simulink model "takeoff_sim"  (R2021b)
settings: Solver=VariableStepAuto  StartTime=0.0  StopTime=5  RelTol=1e-3
values from neighbouring files (symbols this model uses):
  A_cxsec = .0166*1.524 + .014    (= 0.0392984)    [Takeoff_Analysis.m]
  C_do = .03    (= 0.03)    [Takeoff_Analysis.m]
  C_L = 1.4    [Takeoff_Analysis.m]
  g = 9.8    [Takeoff_Analysis.m]
  m = 6.35    [Takeoff_Analysis.m]
  mu = 0.015    [Takeoff_Analysis.m]
  rho = 1.225    [Takeoff_Analysis.m]
  S_cref = 0.46    [Takeoff_Analysis.m]
  S_tref = 0.6    [Takeoff_Analysis.m]
settings Model: Creator=medium boss  LastModifiedBy=medium boss

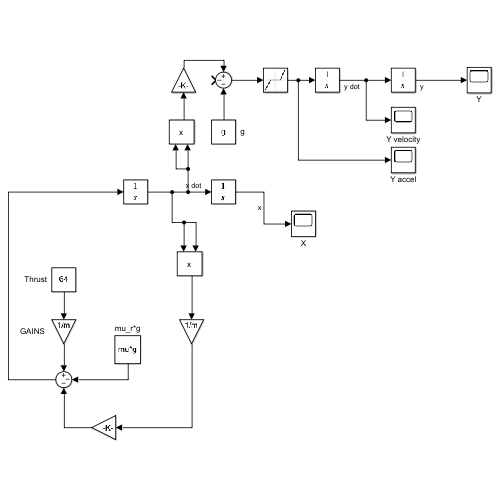
[thumbnail: Simulink's stored preview of the top-level diagram]
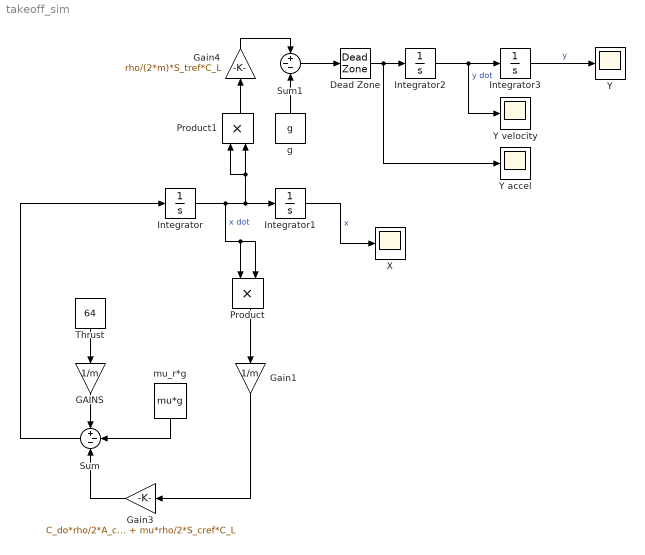
== system takeoff_sim ==
  Dead Zone : DeadZone  LowerValue=-20  UpperValue=0  SaturateOnIntegerOverflow=on
  "GAINS " : Gain  Gain=1/m
  Gain1 : Gain  Gain=1/m
  Gain3 : Gain  Gain=C_do*rho/2*A_cxsec + mu*rho/2*S_cref*C_L
  Gain4 : Gain  Gain=rho/(2*m)*S_tref*C_L
  Integrator{,1..3} (4 alike) : Integrator
  Product : Product
  Product1 : Product
  Sum : Sum  Inputs=+--
  Sum1 : Sum  Inputs=+--
  Thrust : Constant  Value=64
  X : Scope
  Y : Scope
  Y accel : Scope
  Y velocity : Scope
  g : Constant  Value=g
  mu_r*g : Constant  Value=mu*g
  wires:
  Integrator/1 -> Integrator1/1, Product1/1, Product1/2, Product/2, Product/1  "x dot"
  Integrator1/1 -> X/1  "x"
  Product/1 -> Gain1/1
  Thrust/1 -> "GAINS "/1
  "GAINS "/1 -> Sum/1
  mu_r*g/1 -> Sum/2
  Gain3/1 -> Sum/3
  Gain1/1 -> Gain3/1
  Sum/1 -> Integrator/1
  Integrator2/1 -> Y velocity/1, Integrator3/1  "y dot"
  Integrator3/1 -> Y/1  "y"
  g/1 -> Sum1/3
  Product1/1 -> Gain4/1
  Gain4/1 -> Sum1/1
  Sum1/1 -> Dead Zone/1
  Dead Zone/1 -> Y accel/1, Integrator2/1
